simulink subsystem "EFK_correction_multiIMU"  (R2021a)
settings: Solver=VariableStepAuto  StartTime=0.0  StopTime=10.0  RelTol=1e-3
undefined symbols (not defined in the file): acc_std, mag_std, magnitude
libraries: dspmtrx3 x2, attitude_library x2, aerolibutil x1
settings Model: Creator=Laura  LastModifiedBy=Laura

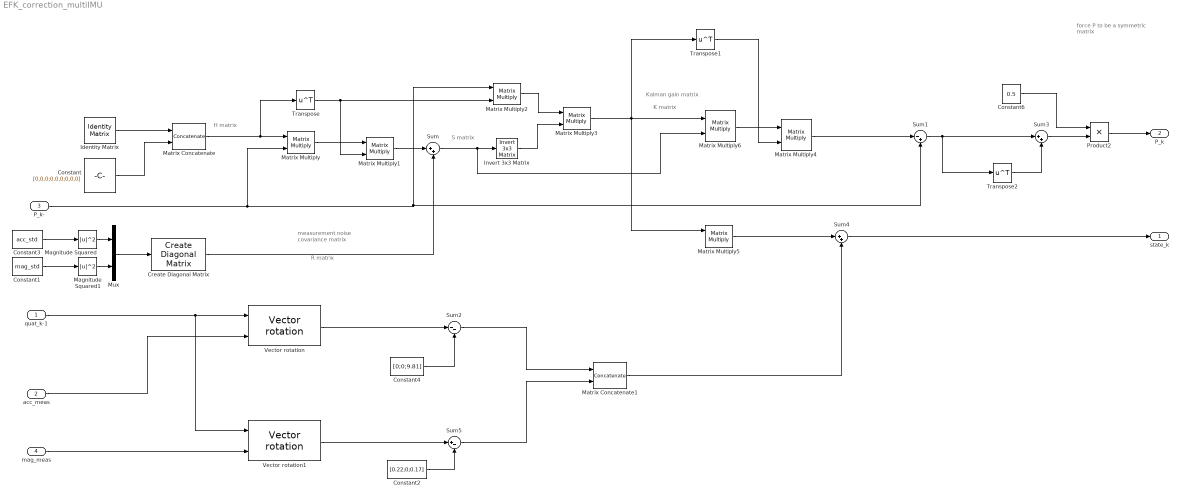
== system EFK_correction_multiIMU ==
  note: measurement noise covariance matrix
  note: H matrix
  note: R matrix
  note: S matrix
  note: K matrix
  note: force P to be a symmetric matrix
  note: Kalman gain matrix
  quat_k-1 : Inport  SampleTime=1/40
  acc_meas : Inport  Port=2  SampleTime=1/40
  P_k- : Inport  Port=3  SampleTime=1/40
  mag_meas : Inport  Port=4  SampleTime=1/40
  Constant : Constant  Value=[0,0,0;0,0,0;0,0,0]
  Constant1 : Constant  Value=mag_std
  Constant2 : Constant  Value=[0.22;0;0.17]
  Constant3 : Constant  Value=acc_std
  Constant4 : Constant  Value=[0;0;9.81]
  Constant6 : Constant  Value=0.5
  Create Diagonal Matrix : dspmtrx3/Create Diagonal Matrix
      settings: SourceProductBaseCode=DS
  Identity Matrix : dspmtrx3/Identity Matrix  Inherit=off  N=3  Ts=1  dataType=double  isSigned=on  wordLen=16  udDataType=sfix(16)  fracBitsMode=Best precision  numFracBits=15  OutDataTypeStr=double  LastOutDataTypeStr=double
  Invert 3x3 Matrix : aerolibutil/Invert  3x3 Matrix
  Magnitude Squared : Math  Operator=magnitude^2  SaturateOnIntegerOverflow=on
  Magnitude Squared1 : Math  Operator=magnitude^2  SaturateOnIntegerOverflow=on
  Matrix Concatenate : Concatenate  Mode=Multidimensional array  ConcatenateDimension=2
  Matrix Concatenate1 : Concatenate  Mode=Multidimensional array
  Matrix Multiply{,1..6} (7 alike) : Product  Multiplication=Matrix(*)
  Mux : Mux  Inputs=2
  Product2 : Product
  Sum : Sum  Inputs=|++
  Sum1 : Sum  Inputs=|-+
  Sum2 : Sum  Inputs=|--
  Sum3 : Sum  Inputs=|++
  Sum4 : Sum  Inputs=|++
  Sum5 : Sum  Inputs=|+-
  Transpose : Math  Operator=transpose  SaturateOnIntegerOverflow=on
  Transpose1 : Math  Operator=transpose  SaturateOnIntegerOverflow=on
  Transpose2 : Math  Operator=transpose  SaturateOnIntegerOverflow=on
  Vector rotation : attitude_library/Vector rotation  SystemSampleTime=-1  VariantActivationTime=update diagram  Latency=0  AutoFrameSizeCalculation=off
      settings: SourceProductName=Attitude library
  Vector rotation1 : attitude_library/Vector rotation  SystemSampleTime=-1  VariantActivationTime=update diagram  Latency=0  AutoFrameSizeCalculation=off
      settings: SourceProductName=Attitude library
  state_k : Outport  SampleTime=1/40
  P_k : Outport  Port=2  SampleTime=1/40
  wires:
  Matrix Multiply3/1 -> Matrix Multiply5/1, Transpose1/1, Matrix Multiply6/1
  Transpose2/1 -> Sum3/2
  Constant6/1 -> Product2/1
  Product2/1 -> P_k/1
  Sum3/1 -> Product2/2
  Invert 3x3 Matrix/1 -> Matrix Multiply3/2
  Matrix Multiply2/1 -> Matrix Multiply3/1
  Matrix Multiply/1 -> Matrix Multiply1/1
  Matrix Multiply1/1 -> Sum/1
  Create Diagonal Matrix/1 -> Sum/2
  Transpose/1 -> Matrix Multiply1/2, Matrix Multiply2/2
  P_k-/1 -> Sum1/2, Matrix Multiply2/1, Matrix Multiply/2
  Matrix Concatenate/1 -> Matrix Multiply/1, Transpose/1
  Constant/1 -> Matrix Concatenate/2
  Identity Matrix/1 -> Matrix Concatenate/1
  Constant3/1 -> Magnitude Squared/1
  Matrix Multiply5/1 -> Sum4/1
  Sum4/1 -> state_k/1
  Sum1/1 -> Sum3/1, Transpose2/1
  Constant1/1 -> Magnitude Squared1/1
  Mux/1 -> Create Diagonal Matrix/1
  Magnitude Squared1/1 -> Mux/2
  Magnitude Squared/1 -> Mux/1
  Sum/1 -> Invert 3x3 Matrix/1, Matrix Multiply6/2
  Matrix Multiply6/1 -> Matrix Multiply4/1
  Transpose1/1 -> Matrix Multiply4/2
  Matrix Multiply4/1 -> Sum1/1
  quat_k-1/1 -> Vector rotation1/1, Vector rotation/1
  acc_meas/1 -> Vector rotation/2
  Vector rotation/1 -> Sum2/1
  Constant4/1 -> Sum2/2
  mag_meas/1 -> Vector rotation1/2
  Vector rotation1/1 -> Sum5/1
  Constant2/1 -> Sum5/2
  Sum2/1 -> Matrix Concatenate1/1
  Sum5/1 -> Matrix Concatenate1/2
  Matrix Concatenate1/1 -> Sum4/2
